simulink model "sim_opencontact"  (R2014a)
settings: Solver=ode14x  StartTime=0.0  StopTime=40e-3  FixedStep=1e-6  RelTol=1e-5
libraries: fl_lib x5, nesl_utility x4, elec_lib x1, ArcLib_lib x1, simulink x1
settings Model: Creator=Dr J  LastModifiedBy=Dr J

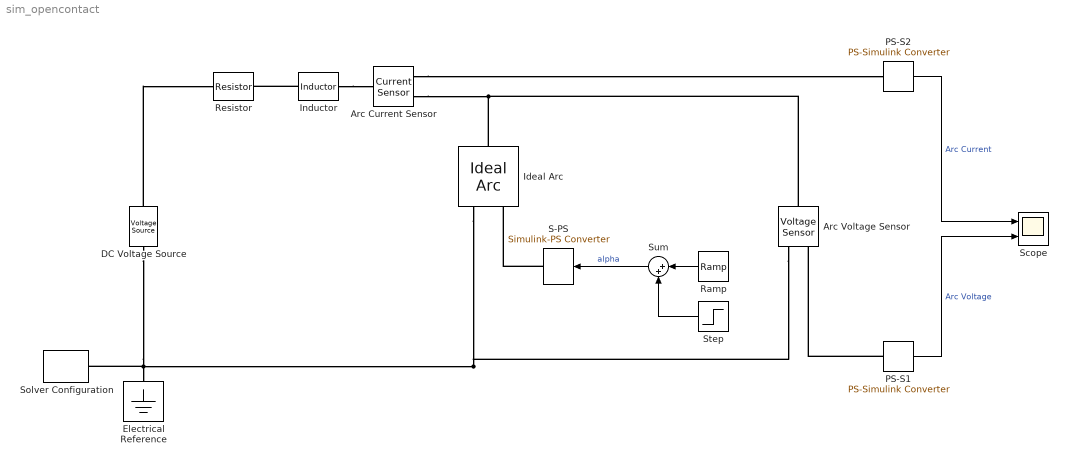
== system sim_opencontact ==
  Arc Current Sensor : fl_lib/Electrical/Electrical Sensors/Current Sensor
  Arc Voltage Sensor : fl_lib/Electrical/Electrical Sensors/Voltage Sensor
  DC Voltage Source : elec_lib/Sources/Voltage Source  dc_voltage=36 V  ac_voltage=0 V  ac_shift=0 deg  ac_frequency=50 Hz  noise_mode=0  PSD=0 V^2/Hz  sample_time=0.001 s  repeatability=1  auto_seed=399384400  user_seed=0
  Electrical Reference : fl_lib/Electrical/Electrical Elements/Electrical Reference
  Ideal Arc : ArcLib_lib/Ideal Arc  b=0.2  Rc=30000 Ohm  TauV=4.5e-5 s  TauI=4.5e-5 s  i_specify=on  i_priority=High  i=300 A  v_specify=on  v_priority=High  v=0.001 V  it_specify=on  it_priority=High  it=1e-4 A
  Inductor : fl_lib/Electrical/Electrical Elements/Inductor  l=0.1e-3 H  r=0 Ohm  g=1e-9 1/Ohm  i_specify=off  i_priority=High  i=300 A  v_specify=off  v_priority=High  v=0 V  i_L_specify=on  i_L_priority=High  i_L=327.27 A
  PS-S1 : nesl_utility/PS-Simulink Converter  PhysicalDomain=network_engine_domain  SubClassName=ps_output  LeftPortType=input  RightPortType=output  PseudoPeriodic=off  Frequencies=[]  Unit=1  AffineConversion=off
  PS-S2 : nesl_utility/PS-Simulink Converter  PhysicalDomain=network_engine_domain  SubClassName=ps_output  LeftPortType=input  RightPortType=output  PseudoPeriodic=off  Frequencies=[]  Unit=1  AffineConversion=off
  Ramp : simulink/Sources/Ramp  slope=1000  start=0.01  X0=0
  Resistor : fl_lib/Electrical/Electrical Elements/Resistor  R=0.11 Ohm  i_specify=off  i_priority=High  i=10 A  v_specify=off  v_priority=High  v=0 V
  S-PS : nesl_utility/Simulink-PS Converter  PhysicalDomain=network_engine_domain  SubClassName=ps_input  LeftPortType=input  RightPortType=output  PseudoPeriodic=off  Frequencies=[]  NoiseDistribution=none  NoiseParameters=[]  Unit=1  AffineConversion=off  InputFiltering=off  SimscapeFilterOrder=1  InputFilterTimeConstant=0.001  UdotUserProvided=1
  Scope : Scope  NumInputPorts=2
      settings: YMin=34.2~0  YMax=37.8~55  SaveName=ScopeData2
  Solver Configuration : nesl_utility/Solver Configuration  PhysicalDomain=network_engine_domain  SubClassName=solver  LeftPortType=input  RightPortType=generic  Accelerate=off  Tones=[]  Harmonics=[]  SimulateNoise=off  Profile=off  UseLocalSampling=off  EnableSwitchedLinearOptims=on  FrequencyDomain=off  UseCCode=off  RelTol=0.001  AbsTol=1e-06  MinStep=1e-09  ToWorkspace=off  DoDC=off  ResidualTolerance=1e-09  UseLocalSolver=on  LocalSolverChoice=NE_BACKWARD_EULER_ADVANCER  LocalSolverSampleTime=1e-6  DoFixedCost=on  MaxNonlinIter=3  MaxModeIter=2  LinearAlgebra=Sparse  DelaysMemoryBudget=1024  AutomaticFiltering=on  FilteringTimeConstant=0.001
  Step : Step  Time=0.01  After=24  SampleTime=0
  Sum : Sum  Inputs=|++
  wires:
  Ramp/1 -> Sum/1
  Sum/1 -> S-PS/1  "alpha"
  Step/1 -> Sum/2
  PS-S2/1 -> Scope/1  "Arc Current"
  PS-S1/1 -> Scope/2  "Arc Voltage"
  connections:
  Electrical Reference/LConn1 -- DC Voltage Source/RConn1 -- Ideal Arc/RConn1 -- Arc Voltage Sensor/RConn2 -- Solver Configuration/RConn1
  DC Voltage Source/LConn1 -- Resistor/LConn1
  Ideal Arc/LConn1 -- Arc Voltage Sensor/LConn1 -- Arc Current Sensor/RConn2
  S-PS/RConn1 -- Ideal Arc/RConn2
  Arc Current Sensor/RConn1 -- PS-S2/LConn1
  PS-S1/LConn1 -- Arc Voltage Sensor/RConn1
  Inductor/LConn1 -- Resistor/RConn1
  Inductor/RConn1 -- Arc Current Sensor/LConn1
